simulink model "ziegler_nichols_PIpseudoD"  (R2026a)
settings: Solver=VariableStepAuto  StopTime=15
values from neighbouring files (symbols this model uses):
  a = 100    [main_root_locus_refinement.m]
  G_den = [1 4 9 10 0]    [main_compare_ziegler_nichols.m]    (also in main_root_locus_refinement.m)
  G_num = [1 -2 10]    [main_compare_ziegler_nichols.m]    (also in main_root_locus_refinement.m)
undefined symbols (not defined in the file or in its folder): KD, KI, KP
settings Model: Creator=nuris  LastModifiedBy=nuris

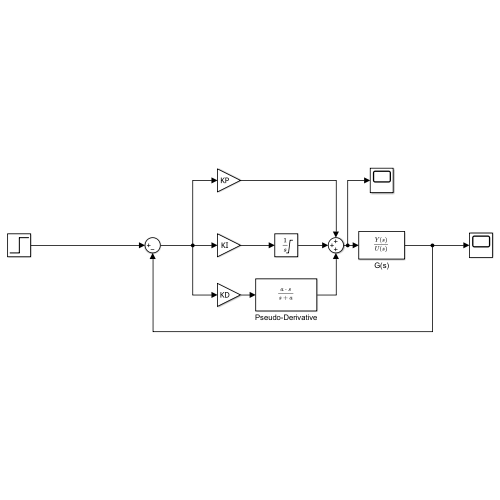
[thumbnail: Simulink's stored preview of the top-level diagram]
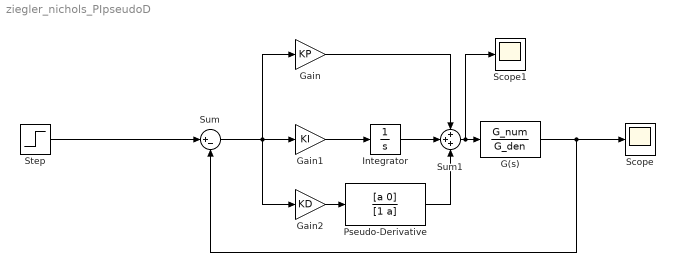
== system ziegler_nichols_PIpseudoD ==
  G(s) : TransferFcn  Numerator=G_num  Denominator=G_den
  Gain : Gain  Gain=KP
  Gain1 : Gain  Gain=KI
  Gain2 : Gain  Gain=KD
  Integrator : Integrator  LimitOutput=on  UpperSaturationLimit=10  LowerSaturationLimit=-2
  Pseudo-Derivative : TransferFcn  Numerator=[a 0]  Denominator=[1 a]
  Scope : Scope
      settings: ActiveDisplayYMinimum=0.23827573483221121  ActiveDisplayYMaximum=2.1999939193430706
  Scope1 : Scope
      settings: ActiveDisplayYMinimum=-7.3373009808058383  ActiveDisplayYMaximum=63.035255664533977
  Step : Step  SampleTime=0
  Sum : Sum  Inputs=|+-
  Sum1 : Sum  Inputs=+++
  wires:
  Step/1 -> Sum/1
  G(s)/1 -> Sum/2, Scope/1
  Gain1/1 -> Integrator/1
  Integrator/1 -> Sum1/2
  Sum1/1 -> Scope1/1, G(s)/1
  Gain/1 -> Sum1/1
  Sum/1 -> Gain/1, Gain2/1, Gain1/1
  Gain2/1 -> Pseudo-Derivative/1
  Pseudo-Derivative/1 -> Sum1/3
